simulink model "AC_1"  (R2022b)
settings: Solver=VariableStepAuto  StartTime=0.0  StopTime=10.0  RelTol=1e-3
libraries: simulink x1
settings Model: Creator=张倬境  LastModifiedBy=张倬境

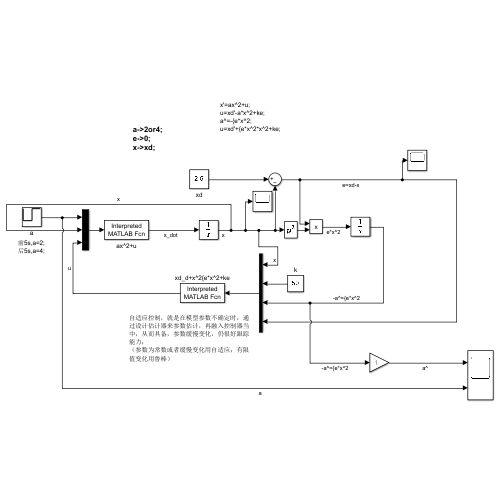
[thumbnail: Simulink's stored preview of the top-level diagram]
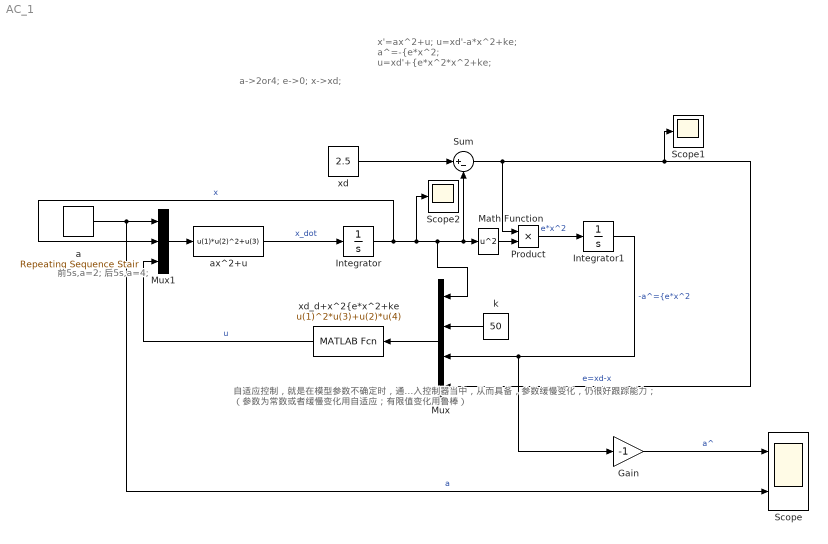
== system AC_1 ==
  note: 自适应控制，就是在模型参数不确定时，通过设计估计器来参数估计，再融入控制器当中，从而具备，参数缓慢变化，仍很好跟踪能力；
      | （参数为常数或者缓慢变化用自适应；有限值变化用鲁棒）
  note: 前5s,a=2;
      | 后5s,a=4;
  note: x'=ax^2+u;
      | u=xd'-a*x^2+ke;
      | a^=-{e*x^2;
      | u=xd'+{e*x^2*x^2+ke;
  note: a->2or4;
      | e->0;
      | x->xd;
  Gain : Gain  Gain=-1
  Integrator : Integrator
  Integrator1 : Integrator
  Math Function : Math  Operator=square
  Mux : Mux
  Mux1 : Mux  Inputs=3
  Product : Product
  Scope : Scope  NumInputPorts=2
  Scope1 : Scope
  Scope2 : Scope
  Sum : Sum  Inputs=|+-
  a : simulink/Sources/Repeating Sequence Stair  OutValues=[2 4]  tsamp=5  OutMin=[]  OutMax=[]  OutDataTypeStr=double  OutputDataTypeScalingMode=double  OutDataType=fixdt(0,8)  ConRadixGroup=Best Precision: Vector-wise  OutScaling=2^-12
  ax^2+u : MATLABFcn  MATLABFcn=u(1)*u(2)^2+u(3)
  k : Constant  Value=50
  xd : Constant  Value=2.5
  "xd_d+x^2{e*x^2+ke" : MATLABFcn  MATLABFcn=u(1)^2*u(3)+u(2)*u(4)
  wires:
  Mux/1 -> "xd_d+x^2{e*x^2+ke"/1
  Integrator/1 -> Scope2/1, Mux/1, Sum/2, Math Function/1, Mux1/2  "x"
  Mux1/1 -> ax^2+u/1
  a/1 -> Scope/2, Mux1/1  "a"
  "xd_d+x^2{e*x^2+ke"/1 -> Mux1/3  "u"
  ax^2+u/1 -> Integrator/1  "x_dot"
  xd/1 -> Sum/1
  Sum/1 -> Product/1, Scope1/1, Mux/4  "e=xd-x"
  Integrator1/1 -> Gain/1, Mux/3  "-a^={e*x^2"
  Math Function/1 -> Product/2
  Product/1 -> Integrator1/1  "e*x^2"
  k/1 -> Mux/2
  Gain/1 -> Scope/1  "a^"
